simulink model "nlplant_testing"  (R2021a)
settings: Solver=FixedStepAuto  StartTime=0.0  StopTime=10.0  FixedStep=0.001  RelTol=1e-3
undefined symbols (not defined in the file or in its folder): dLEF, fi_flag_Simulink, trim_control, trim_state, trim_thrust
settings Model: Creator=johnviljoen  LastModifiedBy=johnviljoen
settings RTWCC: GenCodeOnly=on

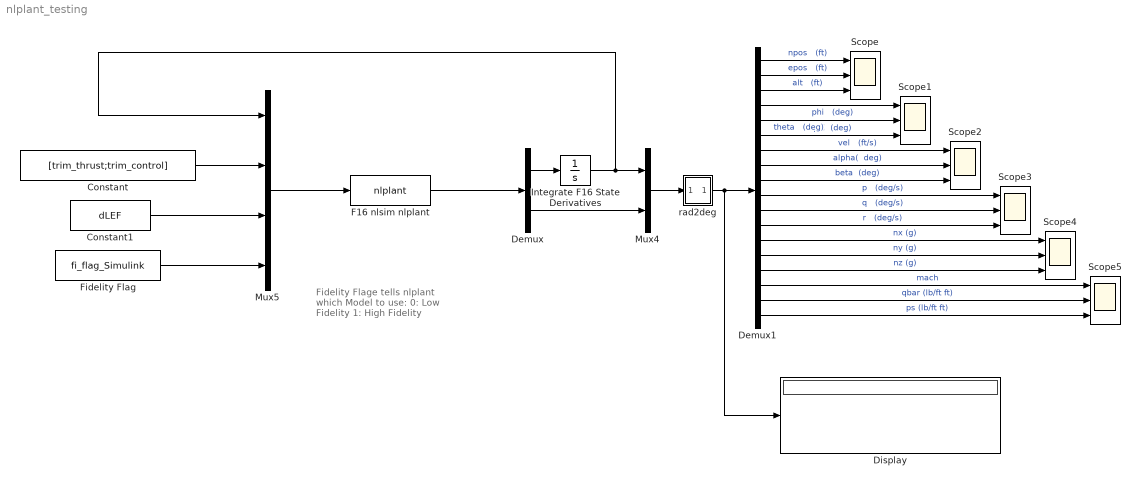
== system nlplant_testing ==
  note: Fidelity Flage tells nlplant
      | which Model to use:
      | 0: Low Fidelity
      | 1: High Fidelity
  Constant : Constant  Value=[trim_thrust;trim_control]
  Constant1 : Constant  Value=dLEF
  Demux : Demux  Outputs=[12 6]
      settings: DisplayOption=none
  Demux1 : Demux  Outputs=18
      settings: DisplayOption=none
  Display : Display
  F16 nlsim nlplant : MATLABFcn  MATLABFcn=nlplant  OutputDimensions=18  OutputSignalType=real
  Fidelity Flag : Constant  Value=fi_flag_Simulink
  Integrate F16 State Derivatives : Integrator  InitialCondition=trim_state
  Mux4 : Mux  Inputs=2
  Mux5 : Mux  Inputs=[12 4 1 1]
  Scope{,1..5} (6 alike) : Scope  NumInputPorts=3
  rad2deg : Subsystem
  wires:
  Integrate F16 State Derivatives/1 -> Mux5/1, Mux4/1
  Fidelity Flag/1 -> Mux5/4
  Mux5/1 -> F16 nlsim nlplant/1
  Constant/1 -> Mux5/2
  F16 nlsim nlplant/1 -> Demux/1
  Mux4/1 -> rad2deg/1(In1)
  Demux/1 -> Integrate F16 State Derivatives/1
  Demux/2 -> Mux4/2
  Constant1/1 -> Mux5/3
  Demux1/10 -> Scope3/1  "p   (deg/s)"
  Demux1/4 -> Scope1/1  "phi   (deg)"
  Demux1/8 -> Scope2/2  "alpha(  deg)"
  Demux1/12 -> Scope3/3  "r   (deg/s)"
  Demux1/13 -> Scope4/1  "nx (g)"
  Demux1/2 -> Scope/2  "epos   (ft)"
  Demux1/16 -> Scope5/1  "mach"
  Demux1/17 -> Scope5/2  "qbar (lb/ft ft)"
  Demux1/7 -> Scope2/1  "vel   (ft/s)"
  Demux1/1 -> Scope/1  "npos   (ft)"
  Demux1/15 -> Scope4/3  "nz (g)"
  rad2deg/1(Out1) -> Display/1, Demux1/1
  Demux1/18 -> Scope5/3  "ps (lb/ft ft)"
  Demux1/14 -> Scope4/2  "ny (g)"
  Demux1/3 -> Scope/3  "alt   (ft)"
  Demux1/9 -> Scope2/3  "beta  (deg)"
  Demux1/11 -> Scope3/2  "q   (deg/s)"
  Demux1/6 -> Scope1/3  "psi  (deg)"
  Demux1/5 -> Scope1/2  "theta   (deg)"

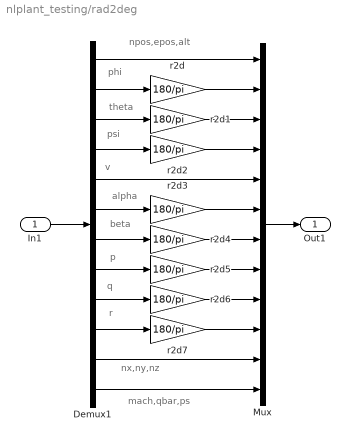
== system nlplant_testing/rad2deg ==
  note: npos,epos,alt
  note: phi
  note: theta
  note: psi
  note: v
  note: alpha
  note: beta
  note: p
  note: q
  note: r
  note: nx,ny,nz
  note: mach,qbar,ps
  In1 : Inport
  Demux1 : Demux  Outputs=[3 1 1 1 1 1 1 1 1 1 3 3]
      settings: DisplayOption=none
  Mux : Mux  Inputs=[3 1 1 1 1 1 1 1 1 1 3 3]
  r2d{,1..7} (8 alike) : Gain  Gain=180/pi  SaturateOnIntegerOverflow=on  OutDataTypeStr=Inherit: Same as input  ParamDataTypeStr=Inherit: Same as input
  Out1 : Outport
  wires:
  In1/1 -> Demux1/1
  Demux1/2 -> r2d/1
  Demux1/3 -> r2d1/1
  Demux1/4 -> r2d2/1
  Demux1/1 -> Mux/1
  Demux1/5 -> Mux/5
  r2d2/1 -> Mux/4
  r2d1/1 -> Mux/3
  r2d/1 -> Mux/2
  Demux1/6 -> r2d3/1
  Demux1/7 -> r2d4/1
  Demux1/8 -> r2d5/1
  Demux1/9 -> r2d6/1
  Demux1/10 -> r2d7/1
  r2d4/1 -> Mux/7
  r2d5/1 -> Mux/8
  r2d6/1 -> Mux/9
  r2d7/1 -> Mux/10
  Mux/1 -> Out1/1
  Demux1/11 -> Mux/11
  Demux1/12 -> Mux/12
  r2d3/1 -> Mux/6
